simulink subsystem "Day4_5_Scenario_1"  (R2024a)
settings: Solver=VariableStepAuto  StartTime=0.0  StopTime=10.0  RelTol=1e-3
libraries: CarMaker4SL x29, robotalgslib x1, matrix_library x1, slpidlib x1
(part 1 of 2)
settings Model: Creator=junhyung.cha  LastModifiedBy=User

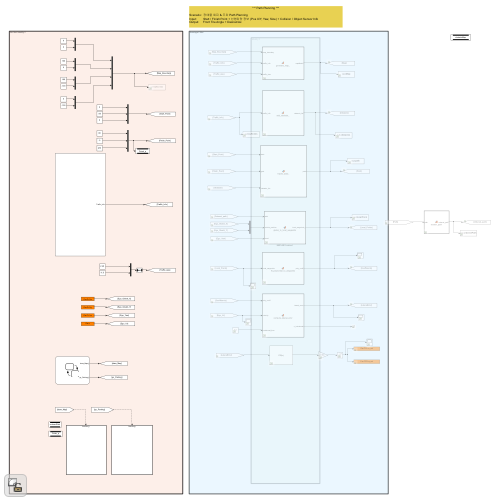
[thumbnail: Simulink's stored preview of the top-level diagram]
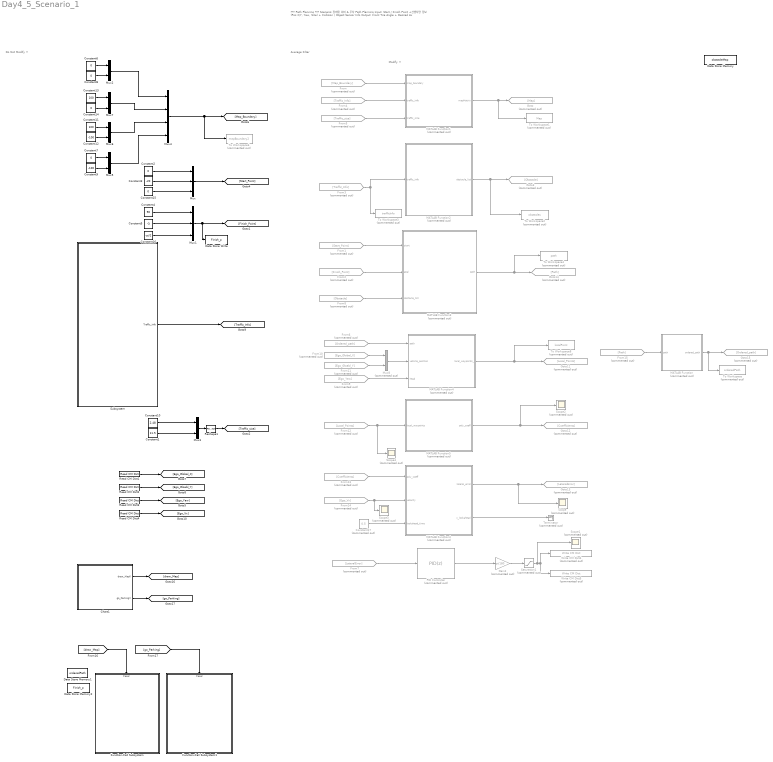
== system Day4_5_Scenario_1 ==
  note: Average Filter
  note: Do Not Modify !!
  note: Modify !!
  note: *** Path Planning ***
      |
      | Scenario: 장애물 회피 & 주차 Path Planning
      | Input: Start / Finish Point + 선행차량 정보 (Pos X/Y, Yaw, Size) + Collision / Object Sensor Info
      | Output: Front Tire Angle + Desired Ax
  Chart1 : Stateflow chart  TreatAsAtomicUnit=on
      settings: PortSchema="{\"entries\":[{\"content\":{\"sides\":[{\"content\":{},\"type\":\"ConnectorPlacement.EquallySpacedRectSide\",\"uuid\":\"919f2d59-559a-485a-ad64-4ca203985945\"},{\"content\":{\"connectorIds\":[\"Out2\",\"Out1\"],\"side\":\"RIGHT\"},\"type\":\"ConnectorPlacement.EquallySpacedRectSide\",\"uuid\":\"5a15d665-f3e4-404a-9c46-468f267f06f6\"},{\"content\":{\"side\":\"TOP\"},\"type\":\"ConnectorPlacement.EquallySpacedRectSide\",\"uuid\":\"06264e3b-ed7f-4ae7-832b-fa30ed2f7930\"}]},\"type\":\"ConnectorPlacement.EquallySpacedConnector\",\"uuid\":\"55c66715-cf4a-4d9b-b78f-cac3e631d511\"}],\"packageUris\":[\"http://schema.mathworks.com/mf0/Connector/R2020b\"],\"version\":\"1.0\"}"
  Constant1 : Constant  Value=11.5
  Constant10 : Constant  Value=2.48
  Constant11 : Constant  Value=100
  Constant12 : Constant  Value=-100
  Constant13 : Constant  Value=100
  Constant{2,6..8,14..15} (6 alike) : Constant  Value=0
  Constant16 : Constant  Value=-pi/2
  Constant17 : Constant  Commented=on  Value=0.5
  Constant3 : Constant  Value=-20
  Constant4 : Constant  Value=90
  Constant5 : Constant  Value=-3
  Constant9 : Constant  Value=-100
  Data Store Memory : DataStoreMemory  DataStoreName=obstacleMap  WriteAfterWriteMsg=warning  VectorParams1D=off  ShowAdditionalParam=off  Dimensions=[70 3]
  Data Store Memory1 : DataStoreMemory  DataStoreName=orderedPath  WriteAfterWriteMsg=warning  ShowAdditionalParam=off  Dimensions=[100 3]
  Data Store Memory2 : DataStoreMemory  DataStoreName=Finish_p  WriteAfterWriteMsg=warning  ShowAdditionalParam=off  Dimensions=[3 1]
  Data Store Write : DataStoreWrite  DataStoreName=Finish_p  IndexOptions=Index vector (dialog)  Indices=1  OutputSizes=1
  From : From  Commented=on  GotoTag=Map_Boundary
  From1 : From  Commented=on  GotoTag=Start_Point
  From10 : From  Commented=on  GotoTag=Ego_Global_X
  From11 : From  Commented=on  GotoTag=Ego_Gloabl_Y
  From12 : From  Commented=on  GotoTag=Local_Points
  From13 : From  Commented=on  GotoTag=Coefficients
  From14 : From  Commented=on  GotoTag=Ego_Vx
  From15 : From  Commented=on  GotoTag=Path
  From2 : From  Commented=on  GotoTag=Finish_Point
  From3 : From  Commented=on  GotoTag=Traffic_Info
  From4 : From  Commented=on  GotoTag=Traffic_Info
  From5 : From  Commented=on  GotoTag=Traffic_size
  From6 : From  Commented=on  GotoTag=Ordered_path
  From7 : From  Commented=on  GotoTag=LateralError
  From8 : From  Commented=on  GotoTag=Obstacle
  From9 : From  Commented=on  GotoTag=Ego_Yaw
  Function-Call Subsystem : Subsystem  TreatAsAtomicUnit=on
  Function-Call Subsystem1 : Subsystem  TreatAsAtomicUnit=on
  Gain2 : Gain  Commented=on  Gain=pi/180
  Goto : Goto  Commented=on  GotoTag=Map
  Goto11 : Goto  Commented=on  GotoTag=Local_Points
  Goto12 : Goto  Commented=on  GotoTag=Coefficients
  Goto13 : Goto  Commented=on  GotoTag=LateralError
  Goto14 : Goto  Commented=on  GotoTag=Path
  Goto15 : Goto  Commented=on  GotoTag=Ordered_path
  Goto3 : Goto  Commented=on  GotoTag=Obstacle
  MATLAB Function : MATLAB Function  Commented=on  TreatAsAtomicUnit=on
  MATLAB Function1 : MATLAB Function  Commented=on  TreatAsAtomicUnit=on
  MATLAB Function2 : MATLAB Function  Commented=on  TreatAsAtomicUnit=on
  MATLAB Function3 : MATLAB Function  Commented=on  TreatAsAtomicUnit=on
  MATLAB Function4 : MATLAB Function  Commented=on  TreatAsAtomicUnit=on
  "MATLAB Function4 " : MATLAB Function  Commented=on  TreatAsAtomicUnit=on
  MATLAB Function5 : MATLAB Function  Commented=on  TreatAsAtomicUnit=on
  Mux : Mux  Inputs=3
  Mux1 : Mux  Inputs=3
  Mux{2..3,5..7} (5 alike) : Mux  Inputs=2
  Mux4 : Mux
  Mux8 : Mux  Commented=on  Inputs=2
  PID Controller : slpidlib/PID Controller  Commented=on  Controller=PID  Form=Parallel  TimeDomain=Discrete-time  UseExternalTs=off  SampleTime=-1  IntegratorMethod=Forward Euler  FilterMethod=Forward Euler  ControllerParametersSource=internal  P=3  I=0  UseKiTs=off  D=0  UseExternalDerivativeSource=off  N=100  UseFilter=on  TunerSelectOption=Transfer Function Based (PID Tuner App)  InitialConditionSource=internal  InitialConditionForIntegrator=0  InitialConditionForFilter=0  DifferentiatorICPrevScaledInput=0  ExternalReset=none  TrackingMode=off  Kt=1  LimitOutput=off  SatLimitsSource=internal  UpperSaturationLimit=inf  LowerSaturationLimit=-inf  LinearizeAsGain=on  AntiWindupMode=none  Kb=1  LimitIntegrator=off  UpperIntegratorSaturationLimit=inf  LowerIntegratorSaturationLimit=-inf  POutMin=[]  POutMax=[]  IOutMin=[]  IOutMax=[]  DOutMin=[]  DOutMax=[]  NOutMin=[]  NOutMax=[]  SumOutMin=[]  SumOutMax=[]  SaturationOutMin=[]  SaturationOutMax=[]  PParamMin=[]  PParamMax=[]  IParamMin=[]  IParamMax=[]  DParamMin=[]  DParamMax=[]  NParamMin=[]  NParamMax=[]  KbParamMin=[]  KbParamMax=[]  KtParamMin=[]  KtParamMax=[]  KbOutMin=[]  KbOutMax=[]  KtOutMin=[]  KtOutMax=[]  IntegratorOutMin=[]  IntegratorOutMax=[]  FilterOutMin=[]  FilterOutMax=[]  SumI1OutMin=[]  SumI1OutMax=[]  SumI2OutMin=[]  SumI2OutMax=[]  SumI3OutMin=[]  SumI3OutMax=[]  SumI4OutMin=[]  SumI4OutMax=[]  SumDOutMin=[]  SumDOutMax=[]  DifferentiatorOutMin=[]  DifferentiatorOutMax=[]  FilterDiffOutCoefMin=[]  FilterDiffOutCoefMax=[]  ReciprocalOutMin=[]  ReciprocalOutMax=[]  SumDenOutMin=[]  SumDenOutMax=[]  SumNumOutMin=[]  SumNumOutMax=[]  DivideOutMin=[]  DivideOutMax=[]  UdiffTsProdOutMin=[]  UdiffTsProdOutMax=[]  NTsProdOutMin=[]  NTsProdOutMax=[]  UintegralTsProdOutMin=[]  UintegralTsProdOutMax=[]  UngainTsProdOutMin=[]  UngainTsProdOutMax=[]  ClampingZeroOutDataTypeStr=Inherit: Inherit via back propagation  ClampingZeroOutMin=[]  ClampingZeroOutMax=[]  FilterDenConstantOutDataTypeStr=Inherit: Inherit via back propagation  FilterDenConstantOutMin=[]  FilterDenConstantOutMax=[]  PCopyOutDataTypeStr=Inherit: Inherit via back propagation  PCopyOutMin=[]  PCopyOutMax=[]  NCopyOutDataTypeStr=Inherit: Inherit via back propagation  NCopyOutMin=[]  NCopyOutMax=[]  IntegratorContinuousStateAttributes=''  IntegratorStateMustResolveToSignalObject=off  IntegratorRTWStateStorageClass=Auto  FilterContinuousStateAttributes=''  FilterStateMustResolveToSignalObject=off  FilterRTWStateStorageClass=Auto  ParallelPVariant=InternalParameters  IdealPVariant=Disabled  IVariant=InternalParameters  DVariant=InternalParameters  IntegratorVariant=Discrete  SatVariant=Disabled  AWVariant=Passthrough  PCopyVariant=Disabled  TRVariant=Disabled  FdbkBlocksVariant=Forward  IdealPFdbkVariant=Disabled  SatFdbkVariant=Disabled  DerivativeFilterVariant=ForwardEulerFilter  NVariant=InternalParameters  NCopyVariant=Disabled  FilterICVariant=InternalICsFilter  IntegratorICVariant=InternalICs  ExternalResetVariant=Disabled  TRSumVariant=Passthrough  SumFdbkVariant=Disabled  SumVariant=Sum_PID  TsampFilterVariant=InternalTs  TsampNgainVariant=Passthrough  TsampIntegralVariant=Disabled_SignalSpec  ExternalSaturationOutDataTypeStr=Inherit: Same as second input  DerivativeSourceVariant=ErrorSignal
  Read CM Dict1 : CarMaker4SL/Read CM Dict  xname=Car.Fr1.tx  xsync=off  xstime=Inherited
  Read CM Dict2 : CarMaker4SL/Read CM Dict  xname=Car.Fr1.ty  xsync=off  xstime=Inherited
  Read CM Dict3 : CarMaker4SL/Read CM Dict  xname=Car.Fr1.rz  xsync=off  xstime=Inherited
  Read CM Dict4 : CarMaker4SL/Read CM Dict  xname=Car.v  xsync=off  xstime=Inherited
  Reshape1 : Reshape  OutputDimensionality=Row vector (2-D)  OutputDimensions=[2,2]
  Saturation1 : Saturate  Commented=on  UpperLimit=2  LowerLimit=-2
  Scope{,1..4} (5 alike) : Scope  Commented=on
  Subsystem : Subsystem
  Terminator : Terminator  Commented=on
  To Workspace : ToWorkspace  Commented=on  VariableName=orderedPath  SampleTime=-1
  To Workspace1 : ToWorkspace  Commented=on  VariableName=Map  SaveFormat=Timeseries  SampleTime=-1
  To Workspace2 : ToWorkspace  Commented=on  VariableName=obstacles  SampleTime=-1
  To Workspace3 : ToWorkspace  Commented=on  VariableName=trafficInfo  SaveFormat=Timeseries  SampleTime=-1
  To Workspace4 : ToWorkspace  Commented=on  VariableName=path  SampleTime=-1
  To Workspace6 : ToWorkspace  Commented=on  VariableName=mapBoundary2  SaveFormat=Timeseries  SampleTime=-1
  To Workspace8 : ToWorkspace  Commented=on  VariableName=localPoint  SampleTime=-1
  Write CM Dict4 : CarMaker4SL/Write CM Dict  Commented=on  xname=Car.CFL.rz_ext  xsync=off
  Write CM Dict5 : CarMaker4SL/Write CM Dict  Commented=on  xname=Car.CFR.rz_ext  xsync=off
  wires:
  Mux/1 -> [Start_Point]
  Constant2/1 -> Mux/1
  Constant3/1 -> Mux/2
  Constant5/1 -> Mux1/2
  Mux1/1 -> [Finish_Point], Data Store Write/1
  Constant4/1 -> Mux1/1
  Constant6/1 -> Mux2/1
  Constant8/1 -> Mux2/2
  Constant9/1 -> Mux5/2
  From/1 -> MATLAB Function1/1(map_boundary)
  Subsystem/1(Traffic_Info) -> [Traffic_Info]
  From3/1 -> MATLAB Function2/1(traffic_info), To Workspace3/1
  Mux3/1 -> Reshape1/1
  Constant10/1 -> Mux3/1
  Constant1/1 -> Mux3/2
  Mux2/1 -> Mux4/1
  Mux5/1 -> Mux4/4
  Mux4/1 -> [Map_Boundary], To Workspace6/1
  Constant7/1 -> Mux5/1
  From4/1 -> MATLAB Function1/2(traffic_info)
  From5/1 -> MATLAB Function1/3(traffic_size)
  Reshape1/1 -> [Traffic_size]
  MATLAB Function1/1(mapMatrix) -> Goto/1, To Workspace1/1
  Read CM Dict4/1 -> [Ego_Vx]
  Read CM Dict1/1 -> [Ego_Global_X]
  Read CM Dict2/1 -> [Ego_Gloabl_Y]
  Read CM Dict3/1 -> [Ego_Yaw]
  Constant11/1 -> Mux6/1
  Constant12/1 -> Mux6/2
  Constant13/1 -> Mux7/1
  Constant14/1 -> Mux7/2
  Mux7/1 -> Mux4/2
  Mux6/1 -> Mux4/3
  Constant15/1 -> Mux/3
  Constant16/1 -> Mux1/3
  MATLAB Function2/1(obstacle_list) -> Goto3/1, To Workspace2/1
  From1/1 -> MATLAB Function3/1(start)
  From2/1 -> MATLAB Function3/2(goal)
  From8/1 -> MATLAB Function3/3(obstacle_list)
  Constant17/1 -> MATLAB Function4/3(lookahead_time)
  From7/1 -> PID Controller/1
  Gain2/1 -> Saturation1/1
  From11/1 -> Mux8/2
  Saturation1/1 -> Write CM Dict4/1, Write CM Dict5/1, Scope1/1
  Mux8/1 -> "MATLAB Function4 "/2(vehicle_position)
  From13/1 -> MATLAB Function4/1(poly_coeff)
  MATLAB Function5/1(poly_coeff) -> Goto12/1, Scope2/1
  MATLAB Function4/1(lateral_error) -> Goto13/1, Scope/1
  MATLAB Function4/2(x_lookahead) -> Terminator/1
  From9/1 -> "MATLAB Function4 "/3(head)
  From12/1 -> MATLAB Function5/1(local_waypoints), Scope4/1
  From10/1 -> Mux8/1
  "MATLAB Function4 "/1(local_waypoints_) -> Goto11/1, To Workspace8/1
  From6/1 -> "MATLAB Function4 "/1(path)
  From14/1 -> MATLAB Function4/2(velocity), Scope3/1
  PID Controller/1 -> Gain2/1
  MATLAB Function3/1(path) -> Goto14/1, To Workspace4/1
  From15/1 -> MATLAB Function/1(path)
  MATLAB Function/1(ordered_path) -> Goto15/1, To Workspace/1
  Chart1/2(draw_Map()) -> [draw_Map]
  [draw_Map] -> Function-Call Subsystem/Trigger
  Chart1/1(go_Parking()) -> [go_Parking]
  [go_Parking] -> Function-Call Subsystem1/Trigger

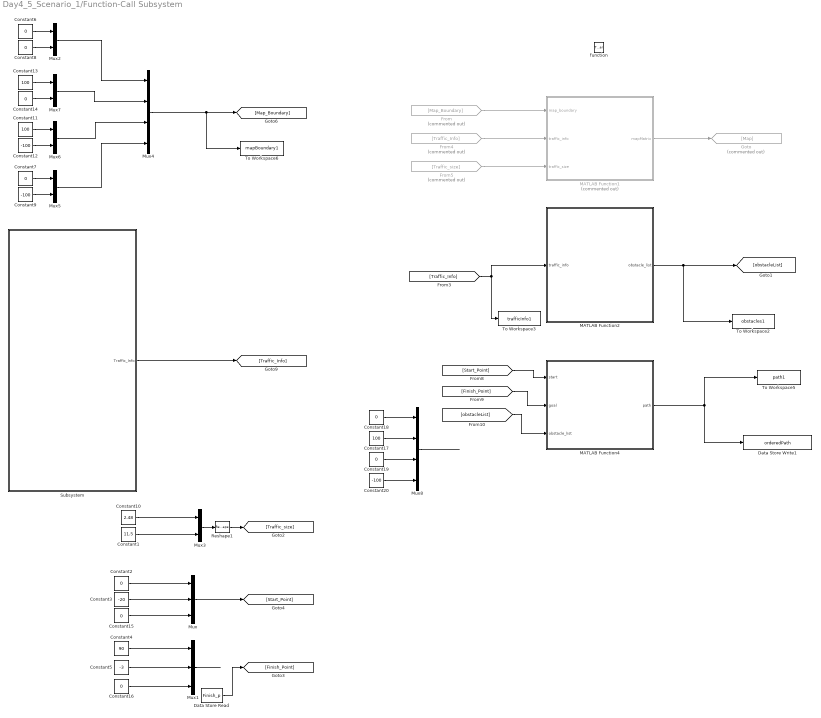
== system Day4_5_Scenario_1/Function-Call Subsystem ==
  function : TriggerPort  TriggerType=function-call  VariantControl=(inherit)
  Constant1 : Constant  Value=11.5
  Constant10 : Constant  Value=2.48
  Constant11 : Constant  Value=100
  Constant12 : Constant  Value=-100
  Constant13 : Constant  Value=100
  Constant{2,6..8,14..16,18..19} (9 alike) : Constant  Value=0
  Constant17 : Constant  Value=100
  Constant20 : Constant  Value=-100
  Constant3 : Constant  Value=-20
  Constant4 : Constant  Value=90
  Constant5 : Constant  Value=-3
  Constant9 : Constant  Value=-100
  Data Store Read : DataStoreRead  DataStoreName=Finish_p  IndexOptions=Index vector (dialog)  Indices=1  OutputSizes=1
  Data Store Write1 : DataStoreWrite  DataStoreName=orderedPath  IndexOptions=Index vector (dialog)  Indices=1  OutputSizes=1
  From : From  Commented=on  GotoTag=Map_Boundary
  From4 : From  Commented=on  GotoTag=Traffic_Info
  From5 : From  Commented=on  GotoTag=Traffic_size
  Goto : Goto  Commented=on  GotoTag=Map
  MATLAB Function1 : MATLAB Function  Commented=on  TreatAsAtomicUnit=on
  MATLAB Function2 : MATLAB Function  TreatAsAtomicUnit=on
  MATLAB Function4 : MATLAB Function  TreatAsAtomicUnit=on
  Mux : Mux  Inputs=3
  Mux1 : Mux  Inputs=3
  Mux{2..3,5..7} (5 alike) : Mux  Inputs=2
  Mux4 : Mux
  Mux8 : Mux
  Reshape1 : Reshape  OutputDimensionality=Row vector (2-D)  OutputDimensions=[2,2]
  Subsystem : Subsystem
  To Workspace2 : ToWorkspace  VariableName=obstacles1  SampleTime=-1
  To Workspace3 : ToWorkspace  VariableName=trafficInfo1  SaveFormat=Timeseries  SampleTime=-1
  To Workspace5 : ToWorkspace  VariableName=path1  SampleTime=-1
      settings: Save2DSignal=2-D array (concatenate along first dimension)
  To Workspace6 : ToWorkspace  VariableName=mapBoundary1  SampleTime=-1
  wires:
  MATLAB Function4/1(path) -> To Workspace5/1, Data Store Write1/1
  Mux8/1 -> ?
  Constant17/1 -> Mux8/2
  Constant18/1 -> Mux8/1
  Constant20/1 -> Mux8/4
  Constant19/1 -> Mux8/3
  [obstacleList] -> MATLAB Function4/3(obstacle_list)
  [Finish_Point] -> MATLAB Function4/2(goal)
  [Start_Point] -> MATLAB Function4/1(start)
  Data Store Read/1 -> [Finish_Point]
  Mux1/1 -> ?
  Constant3/1 -> Mux/2
  Mux/1 -> [Start_Point]
  Constant15/1 -> Mux/3
  Constant5/1 -> Mux1/2
  Constant4/1 -> Mux1/1
  Constant2/1 -> Mux/1
  Constant16/1 -> Mux1/3
  Constant12/1 -> Mux6/2
  MATLAB Function2/1(obstacle_list) -> [obstacleList], To Workspace2/1
  Subsystem/1(Traffic_Info) -> [Traffic_Info]
  Mux5/1 -> Mux4/4
  Mux4/1 -> [Map_Boundary], To Workspace6/1
  [Traffic_Info] -> MATLAB Function2/1(traffic_info), To Workspace3/1
  Constant13/1 -> Mux7/1
  Reshape1/1 -> [Traffic_size]
  Constant1/1 -> Mux3/2
  Constant6/1 -> Mux2/1
  Constant8/1 -> Mux2/2
  From5/1 -> MATLAB Function1/3(traffic_size)
  Constant10/1 -> Mux3/1
  From4/1 -> MATLAB Function1/2(traffic_info)
  Mux6/1 -> Mux4/3
  From/1 -> MATLAB Function1/1(map_boundary)
  Mux3/1 -> Reshape1/1
  Constant7/1 -> Mux5/1
  Constant14/1 -> Mux7/2
  Constant11/1 -> Mux6/1
  Mux2/1 -> Mux4/1
  Mux7/1 -> Mux4/2
  MATLAB Function1/1(mapMatrix) -> Goto/1
  Constant9/1 -> Mux5/2

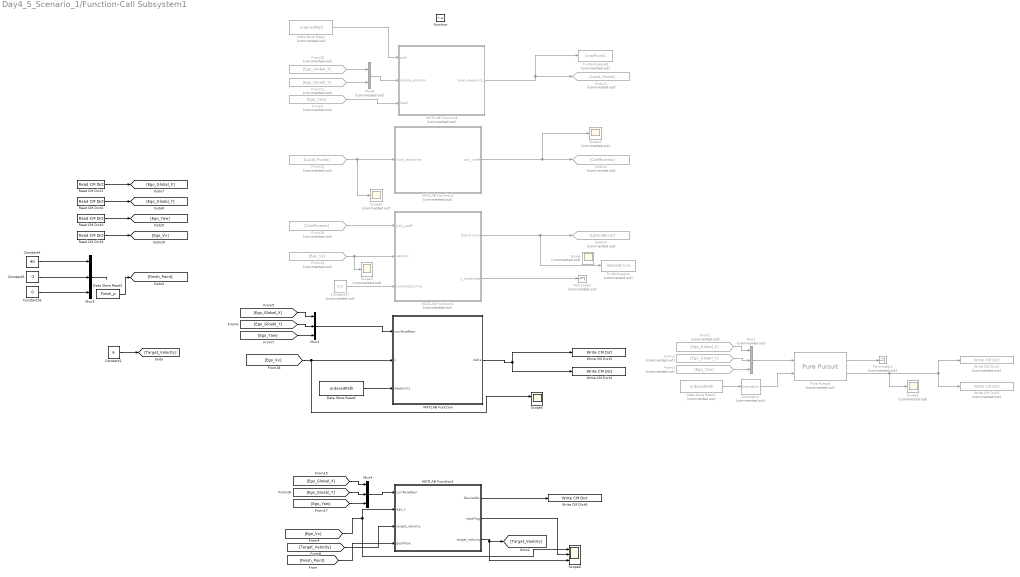
== system Day4_5_Scenario_1/Function-Call Subsystem1 ==
  function : TriggerPort  TriggerType=function-call  VariantControl=(inherit)
  Constant1 : Constant  Value=6
  Constant16 : Constant  Value=0
  Constant17 : Constant  Commented=on  Value=0.5
  Constant4 : Constant  Value=90
  Constant5 : Constant  Value=-3
  Data Store Read : DataStoreRead  Commented=on  DataStoreName=orderedPath  IndexOptions=Index vector (dialog)  Indices=1  OutputSizes=1
  Data Store Read1 : DataStoreRead  Commented=on  DataStoreName=orderedPath  IndexOptions=Index vector (dialog)  Indices=1  OutputSizes=1
  Data Store Read2 : DataStoreRead  DataStoreName=orderedPath  IndexOptions=Index vector (dialog)  Indices=1  OutputSizes=1
  Data Store Read3 : DataStoreRead  DataStoreName=Finish_p  IndexOptions=Index vector (dialog)  Indices=1  OutputSizes=1
  From1 : From  Commented=on  GotoTag=Ego_Global_X
  From10 : From  Commented=on  GotoTag=Ego_Global_X
  From11 : From  Commented=on  GotoTag=Ego_Gloabl_Y
  From12 : From  Commented=on  GotoTag=Local_Points
  From13 : From  Commented=on  GotoTag=Coefficients
  From14 : From  Commented=on  GotoTag=Ego_Vx
  From2 : From  Commented=on  GotoTag=Ego_Gloabl_Y
  From3 : From  Commented=on  GotoTag=Ego_Yaw
  From9 : From  Commented=on  GotoTag=Ego_Yaw
  Goto11 : Goto  Commented=on  GotoTag=Local_Points
  Goto12 : Goto  Commented=on  GotoTag=Coefficients
  Goto13 : Goto  Commented=on  GotoTag=LateralError
  MATLAB Function : MATLAB Function  TreatAsAtomicUnit=on
  MATLAB Function2 : MATLAB Function  TreatAsAtomicUnit=on
  MATLAB Function4 : MATLAB Function  Commented=on  TreatAsAtomicUnit=on
  "MATLAB Function4 " : MATLAB Function  Commented=on  TreatAsAtomicUnit=on
  MATLAB Function5 : MATLAB Function  Commented=on  TreatAsAtomicUnit=on
  Mux1 : Mux  Commented=on  Inputs=3
  Mux2 : Mux  Inputs=3
  Mux3 : Mux  Inputs=3
  Mux4 : Mux  Inputs=3
  Mux8 : Mux  Commented=on  Inputs=2
  Pure Pursuit : robotalgslib/Pure Pursuit  Commented=on  DesiredLinearVelocityPort=off  DesiredLinearVelocity=5  MaxAngularVelocity=2.0  LookaheadDistancePort=off  LookaheadDistance=3  TargetDirPort=off  SimulateUsing=Code generation
  Read CM Dict1 : CarMaker4SL/Read CM Dict  xname=Car.Fr1.tx  xsync=off  xstime=Inherited
  Read CM Dict2 : CarMaker4SL/Read CM Dict  xname=Car.Fr1.ty  xsync=off  xstime=Inherited
  Read CM Dict3 : CarMaker4SL/Read CM Dict  xname=Car.Fr1.rz  xsync=off  xstime=Inherited
  Read CM Dict4 : CarMaker4SL/Read CM Dict  xname=Car.v  xsync=off  xstime=Inherited
  Scope{,1..4} (5 alike) : Scope  Commented=on
  Scope5 : Scope  NumInputPorts=2
  Scope6 : Scope  NumInputPorts=3
  Submatrix : matrix_library/Submatrix  Commented=on  RowSpan=Range of rows  RowStartMode=First  RowStartIndex=1  RowEndMode=Last  RowEndIndex=1  ColSpan=Range of columns  ColStartMode=First  ColStartIndex=1  ColEndMode=Index  ColEndIndex=2
  Terminator : Terminator  Commented=on
  Terminator1 : Terminator  Commented=on
  To Workspace : ToWorkspace  Commented=on  VariableName=lateralErrors  SampleTime=-1
      settings: Save2DSignal=2-D array (concatenate along first dimension)
  To Workspace8 : ToWorkspace  Commented=on  VariableName=localPoint1  SampleTime=-1
  Write CM Dict1 : CarMaker4SL/Write CM Dict  Commented=on  xname=Car.CFL.rz_ext  xsync=off
  Write CM Dict2 : CarMaker4SL/Write CM Dict  Commented=on  xname=Car.CFR.rz_ext  xsync=off
  Write CM Dict3 : CarMaker4SL/Write CM Dict  xname=Car.CFL.rz_ext  xsync=off
  Write CM Dict4 : CarMaker4SL/Write CM Dict  xname=Car.CFR.rz_ext  xsync=off
  Write CM Dict6 : CarMaker4SL/Write CM Dict  xname=AccelCtrl.DesiredAx  xsync=off
  wires:
  Data Store Read3/1 -> [Finish_Point]
  [Ego_Vx] -> MATLAB Function/2(v), Scope5/1
  MATLAB Function2/3(target_velocity) -> [Target_Veolcity], Scope6/3
  [Ego_Yaw] -> Mux4/3
  [Ego_Global_X] -> Mux4/1
  [Ego_Gloabl_Y] -> Mux4/2
  Mux4/1 -> MATLAB Function2/1(currPoseRear)
  MATLAB Function2/2(stopFlag) -> Scope6/2
  Constant1/1 -> [Target_Velocity]
  MATLAB Function2/1(DesiredAx) -> Write CM Dict6/1
  [Ego_Vx] -> MATLAB Function2/2(ego_v), Scope6/1
  [Target_Velocity] -> MATLAB Function2/3("target_velocity ")
  [Finish_Point] -> MATLAB Function2/4(goalPose)
  Constant16/1 -> Mux3/3
  Constant4/1 -> Mux3/1
  Constant5/1 -> Mux3/2
  Mux3/1 -> ?
  Data Store Read2/1 -> MATLAB Function/3(waypoints)
  [Ego_Global_X] -> Mux2/1
  Mux2/1 -> MATLAB Function/1(currPoseRear)
  [Ego_Yaw] -> Mux2/3
  [Ego_Gloabl_Y] -> Mux2/2
  MATLAB Function/1(delta) -> Write CM Dict4/1, Write CM Dict3/1
  Submatrix/1 -> Pure Pursuit/2
  Data Store Read1/1 -> Submatrix/1
  Pure Pursuit/2 -> Write CM Dict2/1, Write CM Dict1/1, Scope1/1
  Pure Pursuit/1 -> Terminator1/1
  From1/1 -> Mux1/1
  From2/1 -> Mux1/2
  From3/1 -> Mux1/3
  Mux1/1 -> Pure Pursuit/1
  Data Store Read/1 -> "MATLAB Function4 "/1(path)
  Read CM Dict2/1 -> [Ego_Gloabl_Y]
  MATLAB Function5/1(poly_coeff) -> Goto12/1, Scope2/1
  Read CM Dict1/1 -> [Ego_Global_X]
  Read CM Dict3/1 -> [Ego_Yaw]
  Read CM Dict4/1 -> [Ego_Vx]
  Mux8/1 -> "MATLAB Function4 "/2(vehicle_position)
  From14/1 -> MATLAB Function4/2(velocity), Scope3/1
  From11/1 -> Mux8/2
  From13/1 -> MATLAB Function4/1(poly_coeff)
  MATLAB Function4/2(x_lookahead) -> Terminator/1
  Constant17/1 -> MATLAB Function4/3(lookahead_time)
  "MATLAB Function4 "/1(local_waypoints_) -> Goto11/1, To Workspace8/1
  From10/1 -> Mux8/1
  From9/1 -> "MATLAB Function4 "/3(head)
  MATLAB Function4/1(lateral_error) -> Goto13/1, To Workspace/1
  From12/1 -> MATLAB Function5/1(local_waypoints), Scope4/1

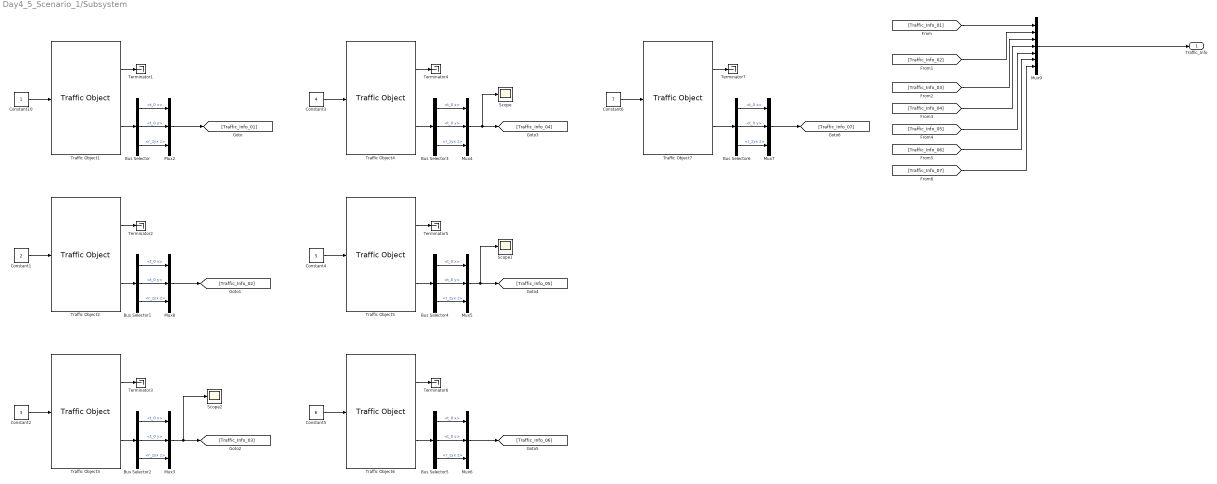
== system Day4_5_Scenario_1/Subsystem ==
  Bus Selector{,1..6} (7 alike) : BusSelector  OutputSignals=t_0 x,t_0 y,r_zyx z
  Constant1 : Constant  Value=2
  Constant10 : Constant
  Constant2 : Constant  Value=3
  Constant3 : Constant  Value=4
  Constant4 : Constant  Value=5
  Constant5 : Constant  Value=6
  Constant6 : Constant  Value=7
  Mux{2..8} (7 alike) : Mux  Inputs=3
  Mux9 : Mux  Inputs=7
  Scope : Scope
  Scope1 : Scope
  Scope2 : Scope
  Terminator{1..7} (7 alike) : Terminator
  Traffic Object1 : CarMaker4SL/Traffic Object  xname=T01  ximode=Traffic Id  xstime=Inherited
      settings: SourceProductName=CarMaker4SL
  Traffic Object2 : CarMaker4SL/Traffic Object  xname=T02  ximode=Traffic Id  xstime=Inherited
      settings: SourceProductName=CarMaker4SL
  Traffic Object3 : CarMaker4SL/Traffic Object  xname=T03  ximode=Traffic Id  xstime=Inherited
      settings: SourceProductName=CarMaker4SL
  Traffic Object4 : CarMaker4SL/Traffic Object  xname=T04  ximode=Traffic Id  xstime=Inherited
      settings: SourceProductName=CarMaker4SL
  Traffic Object5 : CarMaker4SL/Traffic Object  xname=T05  ximode=Traffic Id  xstime=Inherited
      settings: SourceProductName=CarMaker4SL
  Traffic Object6 : CarMaker4SL/Traffic Object  xname=T06  ximode=Traffic Id  xstime=Inherited
      settings: SourceProductName=CarMaker4SL
  Traffic Object7 : CarMaker4SL/Traffic Object  xname=T07  ximode=Traffic Id  xstime=Inherited
      settings: SourceProductName=CarMaker4SL
  Traffic_Info : Outport
  wires:
  [Traffic_Info_07] -> Mux9/7
  [Traffic_Info_06] -> Mux9/6
  [Traffic_Info_05] -> Mux9/5
  [Traffic_Info_04] -> Mux9/4
  [Traffic_Info_03] -> Mux9/3
  Mux9/1 -> Traffic_Info/1
  [Traffic_Info_02] -> Mux9/2
  [Traffic_Info_01] -> Mux9/1
  Mux2/1 -> [Traffic_Info_01]
  Traffic Object7/2 -> Bus Selector6/1
  Bus Selector6/3 -> Mux7/3  "<r_zyx z>"
  Bus Selector6/1 -> Mux7/1  "<t_0 x>"
  Mux7/1 -> [Traffic_Info_07]
  Bus Selector6/2 -> Mux7/2  "<t_0 y>"
  Traffic Object6/2 -> Bus Selector5/1
  Bus Selector5/3 -> Mux6/3  "<r_zyx z>"
  Bus Selector5/1 -> Mux6/1  "<t_0 x>"
  Mux6/1 -> [Traffic_Info_06]
  Bus Selector5/2 -> Mux6/2  "<t_0 y>"
  Traffic Object5/2 -> Bus Selector4/1
  Bus Selector4/3 -> Mux5/3  "<r_zyx z>"
  Bus Selector4/1 -> Mux5/1  "<t_0 x>"
  Mux5/1 -> [Traffic_Info_05], Scope1/1
  Bus Selector4/2 -> Mux5/2  "<t_0 y>"
  Traffic Object4/2 -> Bus Selector3/1
  Bus Selector3/3 -> Mux4/3  "<r_zyx z>"
  Bus Selector3/1 -> Mux4/1  "<t_0 x>"
  Mux4/1 -> [Traffic_Info_04], Scope/1
  Bus Selector3/2 -> Mux4/2  "<t_0 y>"
  Traffic Object3/2 -> Bus Selector2/1
  Bus Selector2/3 -> Mux3/3  "<r_zyx z>"
  Bus Selector2/1 -> Mux3/1  "<t_0 x>"
  Mux3/1 -> [Traffic_Info_03], Scope2/1
  Bus Selector2/2 -> Mux3/2  "<t_0 y>"
  Traffic Object2/2 -> Bus Selector1/1
  Bus Selector1/3 -> Mux8/3  "<r_zyx z>"
  Bus Selector1/1 -> Mux8/1  "<t_0 x>"
  Mux8/1 -> [Traffic_Info_02]
  Bus Selector1/2 -> Mux8/2  "<t_0 y>"
  Bus Selector/3 -> Mux2/3  "<r_zyx z>"
  Bus Selector/2 -> Mux2/2  "<t_0 y>"
  Bus Selector/1 -> Mux2/1  "<t_0 x>"
  Traffic Object1/2 -> Bus Selector/1
  Traffic Object7/1 -> Terminator7/1
  Constant6/1 -> Traffic Object7/1
  Constant5/1 -> Traffic Object6/1
  Traffic Object6/1 -> Terminator6/1
  Traffic Object5/1 -> Terminator5/1
  Constant4/1 -> Traffic Object5/1
  Constant3/1 -> Traffic Object4/1
  Traffic Object4/1 -> Terminator4/1
  Traffic Object3/1 -> Terminator3/1
  Constant2/1 -> Traffic Object3/1
  Constant1/1 -> Traffic Object2/1
  Traffic Object2/1 -> Terminator2/1
  Traffic Object1/1 -> Terminator1/1
  Constant10/1 -> Traffic Object1/1

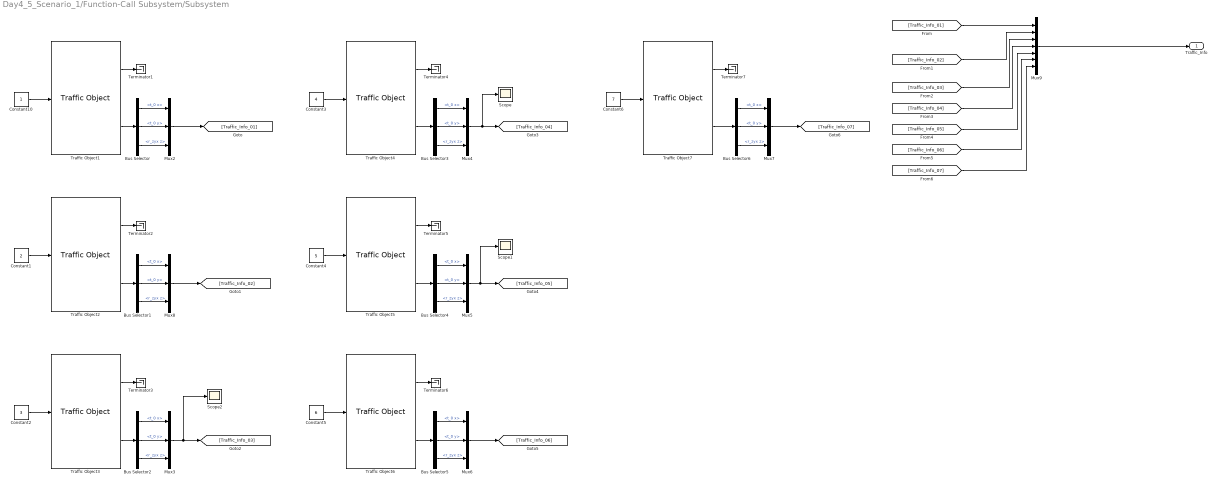
== system Day4_5_Scenario_1/Function-Call Subsystem/Subsystem ==
  Bus Selector{,1..6} (7 alike) : BusSelector  OutputSignals=t_0 x,t_0 y,r_zyx z
  Constant1 : Constant  Value=2
  Constant10 : Constant
  Constant2 : Constant  Value=3
  Constant3 : Constant  Value=4
  Constant4 : Constant  Value=5
  Constant5 : Constant  Value=6
  Constant6 : Constant  Value=7
  Mux{2..8} (7 alike) : Mux  Inputs=3
  Mux9 : Mux  Inputs=7
  Scope : Scope
  Scope1 : Scope
  Scope2 : Scope
  Terminator{1..7} (7 alike) : Terminator
  Traffic Object1 : CarMaker4SL/Traffic Object  xname=T01  ximode=Traffic Id  xstime=Inherited
      settings: SourceProductName=CarMaker4SL
  Traffic Object2 : CarMaker4SL/Traffic Object  xname=T02  ximode=Traffic Id  xstime=Inherited
      settings: SourceProductName=CarMaker4SL
  Traffic Object3 : CarMaker4SL/Traffic Object  xname=T03  ximode=Traffic Id  xstime=Inherited
      settings: SourceProductName=CarMaker4SL
  Traffic Object4 : CarMaker4SL/Traffic Object  xname=T04  ximode=Traffic Id  xstime=Inherited
      settings: SourceProductName=CarMaker4SL
  Traffic Object5 : CarMaker4SL/Traffic Object  xname=T05  ximode=Traffic Id  xstime=Inherited
      settings: SourceProductName=CarMaker4SL
  Traffic Object6 : CarMaker4SL/Traffic Object  xname=T06  ximode=Traffic Id  xstime=Inherited
      settings: SourceProductName=CarMaker4SL
  Traffic Object7 : CarMaker4SL/Traffic Object  xname=T07  ximode=Traffic Id  xstime=Inherited
      settings: SourceProductName=CarMaker4SL
  Traffic_Info : Outport
  wires:
  [Traffic_Info_07] -> Mux9/7
  [Traffic_Info_06] -> Mux9/6
  [Traffic_Info_05] -> Mux9/5
  [Traffic_Info_04] -> Mux9/4
  [Traffic_Info_03] -> Mux9/3
  Mux9/1 -> Traffic_Info/1
  [Traffic_Info_02] -> Mux9/2
  [Traffic_Info_01] -> Mux9/1
  Mux2/1 -> [Traffic_Info_01]
  Traffic Object7/2 -> Bus Selector6/1
  Bus Selector6/3 -> Mux7/3  "<r_zyx z>"
  Bus Selector6/1 -> Mux7/1  "<t_0 x>"
  Mux7/1 -> [Traffic_Info_07]
  Bus Selector6/2 -> Mux7/2  "<t_0 y>"
  Traffic Object6/2 -> Bus Selector5/1
  Bus Selector5/3 -> Mux6/3  "<r_zyx z>"
  Bus Selector5/1 -> Mux6/1  "<t_0 x>"
  Mux6/1 -> [Traffic_Info_06]
  Bus Selector5/2 -> Mux6/2  "<t_0 y>"
  Traffic Object5/2 -> Bus Selector4/1
  Bus Selector4/3 -> Mux5/3  "<r_zyx z>"
  Bus Selector4/1 -> Mux5/1  "<t_0 x>"
  Mux5/1 -> [Traffic_Info_05], Scope1/1
  Bus Selector4/2 -> Mux5/2  "<t_0 y>"
  Traffic Object4/2 -> Bus Selector3/1
  Bus Selector3/3 -> Mux4/3  "<r_zyx z>"
  Bus Selector3/1 -> Mux4/1  "<t_0 x>"
  Mux4/1 -> [Traffic_Info_04], Scope/1
  Bus Selector3/2 -> Mux4/2  "<t_0 y>"
  Traffic Object3/2 -> Bus Selector2/1
  Bus Selector2/3 -> Mux3/3  "<r_zyx z>"
  Bus Selector2/1 -> Mux3/1  "<t_0 x>"
  Mux3/1 -> [Traffic_Info_03], Scope2/1
  Bus Selector2/2 -> Mux3/2  "<t_0 y>"
  Traffic Object2/2 -> Bus Selector1/1
  Bus Selector1/3 -> Mux8/3  "<r_zyx z>"
  Bus Selector1/1 -> Mux8/1  "<t_0 x>"
  Mux8/1 -> [Traffic_Info_02]
  Bus Selector1/2 -> Mux8/2  "<t_0 y>"
  Bus Selector/3 -> Mux2/3  "<r_zyx z>"
  Bus Selector/2 -> Mux2/2  "<t_0 y>"
  Bus Selector/1 -> Mux2/1  "<t_0 x>"
  Traffic Object1/2 -> Bus Selector/1
  Traffic Object7/1 -> Terminator7/1
  Constant6/1 -> Traffic Object7/1
  Constant5/1 -> Traffic Object6/1
  Traffic Object6/1 -> Terminator6/1
  Traffic Object5/1 -> Terminator5/1
  Constant4/1 -> Traffic Object5/1
  Constant3/1 -> Traffic Object4/1
  Traffic Object4/1 -> Terminator4/1
  Traffic Object3/1 -> Terminator3/1
  Constant2/1 -> Traffic Object3/1
  Constant1/1 -> Traffic Object2/1
  Traffic Object2/1 -> Terminator2/1
  Traffic Object1/1 -> Terminator1/1
  Constant10/1 -> Traffic Object1/1

== matlab function Day4_5_Scenario_1/Function-Call Subsystem/MATLAB Function2 ==
  settings: sampleTime=0.1
  data: traffic_info input; obstacle_list output
function obstacle_list = add_obstacle_(traffic_info)
    % 차량 사이즈
    car_w = 2.48;            % 전폭
    car_l = 11.5;            % 전장

    % 장애물 파라미터
    r = car_w / 2 + 2;       % 각 원의 반지름 (1.24 + 2)
    n_circles = 5;          % 각 차량당 원 개수
    interval = car_l / n_circles;  % 원 간격

    % 최대 장애물 개수
    max_obs = 100;
    obstacle_list = zeros(max_obs, 3);  % [x, y, r]

    % === 데이터 복원 ===
    % 데이터가 직렬화된 벡터 형태로 들어오는 경우 처리
    if size(traffic_info, 2) == 1
        % 데이터를 3열 형태로 변환
        n = length(traffic_info) / 3;
        if mod(length(traffic_info), 3) == 0
            % 직렬 데이터를 [N x 3] 행렬로 변환
            latest_data = reshape(traffic_info, 3, n)';  % [N x 3]
            %disp('Reconstructed Data:');
            %disp(latest_data);  % 디버그 출력
        else
            warning('Invalid data length for traffic_info');
            return;
        end
    else
        latest_data = traffic_info;
    end

    % === 데이터 유효성 검사 ===
    if isempty(latest_data) || size(latest_data, 2) < 3
        warning('Latest data is empty or has incorrect dimensions');
        return;
    end

    % 중복 제거: unique 함수 사용 가능 여부 확인
    if size(latest_data, 1) > 1
        % unique 함수로 중복 좌표 제거
        [~, unique_indices] = unique(latest_data(:, 1:2), 'rows', 'stable');
        unique_data = latest_data(unique_indices, :);
    else
        % 데이터가 하나만 있는 경우 그대로 사용
        unique_data = latest_data;
    end

    % 입력 데이터 유효성 검사 및 reshape 처리
    unique_data = reshape(unique_data, [], 3);  % [N x 3]
    [n_rows, ~] = size(unique_data);

    % 장애물 좌표 생성
    count = 0;
    for i = 1:n_rows
        x_head = unique_data(i, 1);
        y_head = unique_data(i, 2);
        yaw = unique_data(i, 3);  % 각도(rad)

        % Yaw 값 검증
        if isnan(yaw) || ~isfinite(yaw)
            yaw = 0;
        end

        % 장애물 생성 (차량의 길이 방향으로)
        for j = 0:n_circles-1
            dx = cos(yaw) * (j * interval);
            dy = sin(yaw) * (j * interval);
            xc = x_head + dx;
            yc = y_head + dy;

            count = count + 1;
            if count <= max_obs
                obstacle_list(count, :) = [xc, yc, r];
            else
                break;
            end
        end
    end

    % 디버그: 결과 확인
    %disp('Generated Obstacle List:');
    %disp(obstacle_list);
    disp("generate_Map_Finish");
end

== matlab function Day4_5_Scenario_1/MATLAB Function ==
  data: path input; ordered_path output
function ordered_path = reorder_path(path)
    %#codegen
    % 입력: path (100x3) - 역순 경로
    % 출력: ordered_path (100x3) - 정순 경로

    % 고정 크기 배열 선언 (100x3)
    ordered_path = NaN(100, 3);  
    
    % 유효 경로 필터링 (NaN 값 제거)
    valid_idx = ~isnan(path(:, 1)) & ~isnan(path(:, 2)) & ~isnan(path(:, 3));
    valid_path = path(valid_idx, :);

    % 유효 경로 개수
    num_points = size(valid_path, 1);

    % 역순으로 배열 채우기 (고정 크기 유지)
    for i = 1:num_points
        ordered_path(i, :) = valid_path(num_points - i + 1, :);
    end

    % 나머지 부분 NaN으로 채우기
    if num_points < 100
        ordered_path((num_points+1):100, :) = NaN;
    end
end

== matlab function Day4_5_Scenario_1/MATLAB Function1 ==
  settings: sampleTime=0.05
  data: map_boundary input; mapMatrix output size=[1000, 1000]; traffic_info input; traffic_size input
% map_boundary = [0, 0, 100, 0, 100, -100, 0, -100];  % 시계방향 사각형
% traffic_info = [
%     40   -12   pi/2;
%     40   -24   pi/2;
%     40   -36   pi/2;
%     40   -48   pi/2;
%     39   -50   0;
%     51   -50   0;
%     63   -50   0];  % [x_head, y_head, yaw]
% traffic_size = [2.48, 11.5];    % [width, length] (m)
% start_point  = [0, -20];
% finish_point = [80, -3];
% 
% a = generate_map_(map_boundary, traffic_info, traffic_size);

function mapMatrix = generate_map_(map_boundary, traffic_info, traffic_size)
%#codegen
% 맵 바운더리 + 장애물 테두리를 마스킹하는 함수
% Y축 반전 처리만 적용 (Y는 -100~0 → mapMatrix는 1~100)

    % === 초기화 ===
    mapMatrix = zeros(100, 100);

    % === reshape 및 파라미터 ===
    traffic_info = reshape(traffic_info, [], 3);  % [N x 3]
    num_traffic = size(traffic_info, 1);
    width  = traffic_size(1);
    length = traffic_size(2);

    % === 장애물 테두리 처리 ===
    for i = 1:num_traffic
        x_head = traffic_info(i,1);
        y_head = traffic_info(i,2);
        yaw    = traffic_info(i,3);
       
        % 머리 좌표를 중심 기준으로 사용
        xc = x_head;
        yc = y_head;

        dx = width / 2;
        dy = length;
        local = [
            0, -dx;
            0,  dx;
            dy, dx;
            dy, -dx
        ];

        R = [cos(yaw), -sin(yaw); sin(yaw), cos(yaw)];
        global_pts = zeros(5, 2);  % 4개 꼭짓점 + 첫 점
        
        global_pts(1:4, :) = (R * local')' + [xc, yc];
        global_pts(5, :)   = global_pts(1, :);  % 꼭짓점 닫기

        for k = 1:4
            x1 = global_pts(k,1);   y1 = global_pts(k,2);
            x2 = global_pts(k+1,1); y2 = global_pts(k+1,2);
            N = 100;
            xs = linspace(x1, x2, N);
            ys = linspace(y1, y2, N);
            for j = 1:N
                x_idx = round(xs(j));
                y_idx = round(-ys(j));  % ✅ Y 좌표 반전

                % 인덱스 클리핑
                x_idx = min(max(x_idx, 1), 100);
                y_idx = min(max(y_idx, 1), 100);

                mapMatrix(y_idx, x_idx) = 1;
            end
        end
    end

    % === 바운더리 테두리 처리 ===
    xb = map_boundary(1:2:end);
    yb = map_boundary(2:2:end);
    xb(end+1) = xb(1);
    yb(end+1) = yb(1);
    for k = 1:4
        x1 = xb(k);   y1 = yb(k);
        x2 = xb(k+1); y2 = yb(k+1);
        N = 100;
        xs = linspace(x1, x2, N);
        ys = linspace(y1, y2, N);
        for j = 1:N
            x_idx = round(xs(j));
            y_idx = round(-ys(j));  % ✅ Y 좌표 반전

            % 인덱스 클리핑
            x_idx = min(max(x_idx, 1), 100);
            y_idx = min(max(y_idx, 1), 100);

            mapMatrix(y_idx, x_idx) = 1;
        end
    end
end

== matlab function Day4_5_Scenario_1/MATLAB Function2 ==
  settings: sampleTime=0.1
  data: traffic_info input; obstacle_list output
function obstacle_list = add_obstacle_(traffic_info)
    % 차량 사이즈
    car_w = 2.48;            % 전폭
    car_l = 11.5;            % 전장

    % 장애물 파라미터
    r = car_w / 2 + 2;       % 각 원의 반지름 (1.24 + 2)
    n_circles = 10;          % 각 차량당 원 개수
    interval = car_l / n_circles;  % 원 간격

    % 최대 장애물 개수
    max_obs = 70;
    obstacle_list = zeros(max_obs, 3);  % [x, y, r]

    % === 데이터 복원 ===
    % 데이터가 직렬화된 벡터 형태로 들어오는 경우 처리
    if size(traffic_info, 2) == 1
        % 데이터를 3열 형태로 변환
        n = length(traffic_info) / 3;
        if mod(length(traffic_info), 3) == 0
            % 직렬 데이터를 [N x 3] 행렬로 변환
            latest_data = reshape(traffic_info, 3, n)';  % [N x 3]
            %disp('Reconstructed Data:');
            %disp(latest_data);  % 디버그 출력
        else
            warning('Invalid data length for traffic_info');
            return;
        end
    else
        latest_data = traffic_info;
    end

    % === 데이터 유효성 검사 ===
    if isempty(latest_data) || size(latest_data, 2) < 3
        warning('Latest data is empty or has incorrect dimensions');
        return;
    end

    % 중복 제거: unique 함수 사용 가능 여부 확인
    if size(latest_data, 1) > 1
        % unique 함수로 중복 좌표 제거
        [~, unique_indices] = unique(latest_data(:, 1:2), 'rows', 'stable');
        unique_data = latest_data(unique_indices, :);
    else
        % 데이터가 하나만 있는 경우 그대로 사용
        unique_data = latest_data;
    end

    % 입력 데이터 유효성 검사 및 reshape 처리
    unique_data = reshape(unique_data, [], 3);  % [N x 3]
    [n_rows, ~] = size(unique_data);

    % 장애물 좌표 생성
    count = 0;
    for i = 1:n_rows
        x_head = unique_data(i, 1);
        y_head = unique_data(i, 2);
        yaw = unique_data(i, 3);  % 각도(rad)

        % Yaw 값 검증
        if isnan(yaw) || ~isfinite(yaw)
            yaw = 0;
        end

        % 장애물 생성 (차량의 길이 방향으로)
        for j = 0:n_circles-1
            dx = cos(yaw) * (j * interval);
            dy = sin(yaw) * (j * interval);
            xc = x_head + dx;
            yc = y_head + dy;

            count = count + 1;
            if count <= max_obs
                obstacle_list(count, :) = [xc, yc, r];
            else
                break;
            end
        end
    end

    % 디버그: 결과 확인
    %disp('Generated Obstacle List:');
    %disp(obstacle_list);
end

== matlab function Day4_5_Scenario_1/Function-Call Subsystem1/MATLAB Function4 ==
  settings: sampleTime=0.05
  data: poly_coeff input; lateral_error output; velocity input; lookahead_time input; x_lookahead output
function [lateral_error, x_lookahead] = compute_lateral_error(poly_coeff, velocity, lookahead_time)
    
    % Lookahead 지점 계산
    x_lookahead = velocity * lookahead_time;
    % 경로 상의 lookahead 지점에서의 y값 계산
    y_desired = polyval(poly_coeff, x_lookahead);

    % lateral error : 차량 y=0 위치와 경로 y_desired의 차이
    lateral_error = y_desired;
end

== matlab function Day4_5_Scenario_1/Function-Call Subsystem1/MATLAB Function4  ==
  settings: sampleTime=0.05
  data: path input; local_waypoints_ output; vehicle_position input; head input
function local_waypoints_ = global_to_local_waypoints(path, vehicle_position, head)
    %#codegen
    % 글로벌 경로를 로컬 경로로 변환해주는 함수
    % path : [x, y, yaw] (경로 점들)
    % vehicle_position : [Ego_Global_X, Ego_Global_Y]
    % head : Ego_Yaw (rad)
    % 출력: 로컬 좌표 (x_local, y_local, yaw_local)

    % 최대 경로 점 개수 설정
    max_points = 100;

    % 초기화
    local_waypoints_ = NaN(max_points, 3);  % 고정 크기 배열

    % 차량 위치 및 헤딩 추출
    ego_x = vehicle_position(1);
    ego_y = vehicle_position(2);
    ego_yaw = head;

    % 회전 행렬 생성 (글로벌→로컬 변환)
    R = [cos(-ego_yaw) -sin(-ego_yaw); 
         sin(-ego_yaw)  cos(-ego_yaw)];

    count = int32(0);  % 경로 점 개수

    % 각 경로 포인트에 대해 변환 수행
    for i = 1:min(size(path, 1), max_points)
        % 글로벌 좌표에서 차량까지의 상대 위치
        dx = path(i, 1) - ego_x;  % X 좌표 차이
        dy = path(i, 2) - ego_y;  % Y 좌표 차이

        % 회전 변환 적용
        local_pos = R * [dx; dy];
        
        % Yaw 변환: 로컬 좌표계에서의 Yaw
        global_yaw = path(i, 3);
        local_yaw = wrapToPi(global_yaw - ego_yaw);  % 로컬 yaw 변환

        % 차량으로부터 waypoint까지의 거리
        distance = sqrt(local_pos(1)^2 + local_pos(2)^2);

        % 첫 번째 유효 경로 점 저장 (x > 0인 첫 포인트)
        if count == 0 && local_pos(1) > 0
            count = count + 1;
            local_waypoints_(count, :) = [local_pos(1), local_pos(2), local_yaw];
        end
        
        % 고정 크기 초과 방지
        if count < max_points
            count = count + 1;
            local_waypoints_(count, :) = [local_pos(1), local_pos(2), local_yaw];
        else
            warning('Maximum number of waypoints reached.');
            break;
        end
    end

    % 남은 부분을 NaN으로 채움
    if count < max_points
        local_waypoints_((count+1):max_points, :) = NaN;
    end
end

== matlab function Day4_5_Scenario_1/Function-Call Subsystem1/MATLAB Function5 ==
  settings: sampleTime=0.05
  data: local_waypoints input; poly_coeff output
function poly_coeff = fit_polynomial_to_waypoints(local_waypoints)
    % waypoint를 curve fitting 한 다항식 계수 반환
    % input: 로컬 좌표 웨이포인트
    % output: 다항식 계수 (3차)

    % 웨이포인트 추출
    x_points = local_waypoints(:, 1);  % 로컬 x 좌표
    y_points = local_waypoints(:, 2);  % 로컬 y 좌표

    % 유효한 웨이포인트만 사용 (x 좌표가 양수인 것만)
    valid_indices = x_points > 0;
    x_valid = x_points(valid_indices);
    y_valid = y_points(valid_indices);

    % 웨이포인트가 충분한지 확인
    if length(x_valid) < 4
        % 웨이포인트가 부족하면 직선 경로 반환
        poly_coeff = [0, 0, 0, 0];  % y = 0 (직선)
    else
        % 3차 다항식 피팅 (y = ax^3 + bx^2 + cx + d)
        poly_coeff = polyfit(x_valid, y_valid, 3);
    end
end

== matlab function Day4_5_Scenario_1/Function-Call Subsystem1/MATLAB Function2 ==
  settings: sampleTime=0.05
  data: currPoseRear input; DesiredAx output; ego_v input; target_velocity input; goalPose input; stopFlag output; target_velocity output
function [DesiredAx,stopFlag,target_velocity] = longitudinal_goal_controller(currPoseRear, ego_v,target_velocity,goalPose)
%▴ 종방향 속도 제어 및 목표 도달 확인
% Inputs:
%   currPoseRear: [x_rear; y_rear; psi] (후륜축 기준)
%   v           : 속도 (m/s)
%   goalPose    : [x_goal; y_goal; psi_goal]
% Outputs:
%   DesiredAx   : 원하는 가속도 (m/s^2)
%   stopFlag    : 목표 도달 시 true

    persistent Kp Kd dt prev_error
  if isempty(Kp)
    % — PD 게인 설정 (필요에 따라 조정하세요) —
    Kp = 1.8;    % 비례 이득
    Kd = 0.1;    % 미분 이득
    % — 제어 업데이트 주기 (Simulink 샘플타임과 동일하게) —
    dt = 0.1;    % [s]
    % — previous error 초기화 —
    prev_error = target_velocity - ego_v;
  end

  % 1) 속도 오차
  error = target_velocity - ego_v;
  % 2) 오차 변화율 (미분항)
  derivative = (error - prev_error) / dt;
  % 3) PD 제어 법칙
  DesiredAx = Kp * error + Kd * derivative;
  % 4) 이전 오차 갱신
  prev_error = error;


    %#codegen
    % 1) 위치·헤딩 오차 계산
    dx     = currPoseRear(1) - goalPose(1);
    dy     = currPoseRear(2) - goalPose(2);
    dist   = hypot(dx, dy);                                           % 거리 계산 :contentReference[oaicite:3]{index=3}
    yawErr = wrapToPi(goalPose(3) - currPoseRear(3));                 % –π~π 범위 :contentReference[oaicite:4]{index=4}

    % 2) 목표 도달 여부 판단 (Goal Checking in Parking Valet) :contentReference[oaicite:5]{index=5}
    posTol = 1.7;             % 위치 허용 오차 [m]
    yawTol = deg2rad(30);     % 헤딩 허용 오차 [rad]
    almostFlag = dist<12;
    distFlag = dist <= posTol;
    yawFlag = abs(yawErr) <= yawTol;
    stopFlag = distFlag && yawFlag;

    % 3) DesiredAx 계산
    if stopFlag
        DesiredAx = -1000;
        disp("stopFlag")% 도착 시 완전 정지
    elseif almostFlag
        target_velocity = 3;
        disp("almost goal")% 근접 시 제동 가속도
        error      = target_velocity - ego_v;
        derivative = (error - prev_error)/dt;
        DesiredAx  = Kp*error + Kd*derivative;
        prev_error = error;
    end
end

== matlab function Day4_5_Scenario_1/MATLAB Function3 ==
  data: start input; path output double size=[100, 3]; goal input; obstacle_list input double size=[70, 3]
function path = hybrid_astar_(start, goal, obstacle_list)
%#codegen

% 기본 파라미터 설정
R = 4;
Vx = 3;
delta_time_step = 1;
weight = 1.3;
space = [0, 100, -100, 0];
res_dijkstra = 1;

% 경로 배열 초기화 (고정 크기)
path = NaN(100, 3);  % 고정 크기 배열
path_count = int32(0);

% 구조체 초기화 함수
default_node = struct('position', zeros(1,3), 'heading', 0.0, 'g', 0.0, 'h', 0.0, 'f', 0.0, 'parent', int32(0));
open_list = repmat(default_node, 1, 100);
closed_list = repmat(default_node, 1, 10000);

% Dijkstra를 이용한 비용 맵 생성
cost_map = run_dijkstra(goal, obstacle_list, space, res_dijkstra);
start_node = create_node(int32(0), start);
goal_node = create_node(int32(0), goal);

% 초기화
open_list(1) = start_node;
open_count = int32(1);
closed_count = int32(0);

% Hybrid A* 알고리즘
while open_count > 0
    % 최저 비용 노드 선택
    f_values = arrayfun(@(n) n.f, open_list(1:open_count));
    [~, idx] = min(f_values);
    temp_node = open_list(idx);
    open_list(idx) = open_list(open_count);
    open_count = open_count - 1;
    closed_count = closed_count + 1;
    closed_list(closed_count) = temp_node;

    % 목표 도달 확인
    if isSamePosition(temp_node, goal_node, 5)
        % 역순으로 경로 저장
        idx = 1;  % 경로 인덱스 초기화
        while temp_node.parent > 0 && path_count < 100
            path_count = path_count + 1;
            % 경로를 역순으로 저장하여 고정 크기 유지
            path(path_count, :) = temp_node.position;
            parent_idx = temp_node.parent;
            temp_node = closed_list(parent_idx);  
            idx = idx + 1;
        end
        % 경로 배열 크기를 고정하여 반환
        if path_count < 100
            path((path_count+1):100, :) = NaN;  % 나머지 부분을 NaN으로 채움
        end
        return;
    end

    % 가능한 액션 생성 및 탐색
    actions = get_action(R, Vx, delta_time_step);
    for i = 1:size(actions, 1)
        yaw_rate = actions(i, 1);
        dt = actions(i, 2);
        new_pos = vehicle_move(temp_node.position, yaw_rate, dt, Vx);
        
        % 탐색 공간 확인 및 충돌 검사
        if isNotInSearchingSpace(new_pos, space), continue; end
        if collision_check(temp_node.position, yaw_rate, dt, obstacle_list, Vx, space), continue; end
        
        % 자식 노드 생성
        child_node = create_node(closed_count, new_pos);
        if any(arrayfun(@(n) isSamePosition(n, child_node, 5) && isSameYaw(n, child_node, 0.3), closed_list(1:closed_count))), continue; end
        
        % 비용 계산
        yaw_diff = abs(angdiff(temp_node.heading, child_node.heading));
        turn_penalty = 2 * yaw_diff;
        child_node.g = temp_node.g + Vx * dt + turn_penalty;
        child_node.h = heuristic(child_node, goal_node, cost_map, space, res_dijkstra);
        child_node.f = child_node.g + weight * child_node.h;

        % 중복 노드 체크
        skip = false;
        for j = 1:open_count
            temp_open = open_list(j);
            if isSamePosition(temp_open, child_node, 5) && child_node.f >= temp_open.f
                skip = true; break;
            end
        end
        if skip, continue; end

        % 오픈 리스트에 추가
        open_count = open_count + 1;
        open_list(open_count) = child_node;
    end
end
% 경로 크기 고정으로 반환
path = path(1:100, :);
end

% 노드 생성 함수
function node = create_node(parent, position)
    % 구조체 필드 초기화 고정
    node = struct('position', zeros(1,3), 'heading', 0.0, 'g', 0.0, 'h', 0.0, 'f', 0.0, 'parent', int32(parent));
    node.position = reshape(position, [1,3]);  % 강제로 크기 고정
    node.heading = position(3);
end

function h = heuristic(cur_node, goal_node, cost_map, space, res)
    gx = round((cur_node.position(1) - space(1)) / res) + 1;
    gy = round((cur_node.position(2) - space(3)) / res) + 1;
    [ny, nx] = size(cost_map);
    if gx < 1 || gx > nx || gy < 1 || gy > ny, h = 1e6; return; end
    cost_dijkstra = cost_map(gy, gx);
    dyaw = abs(angdiff(cur_node.heading, goal_node.heading));
    h = cost_dijkstra + 3 * dyaw;
end

function cost_map = run_dijkstra(goal, obstacle_list, space, res)
x_range = space(1):res:space(2);
y_range = space(3):res:space(4);
nx = length(x_range); ny = length(y_range);
cost_map = inf(ny, nx); visited = false(ny, nx);
gx = round((goal(1) - space(1)) / res) + 1;
gy = round((goal(2) - space(3)) / res) + 1;
cost_map(gy, gx) = 0;

% Preallocate the queue with a fixed size
q = zeros(10000, 2);
q_count = 1;
q(1, :) = [gx, gy];

while q_count > 0
    [~, idx] = min(cost_map(sub2ind(size(cost_map), q(1:q_count,2), q(1:q_count,1))));
    current = q(idx, :);
    q(idx, :) = q(q_count, :);
    q_count = q_count - 1;
    x = current(1); y = current(2);
    if visited(y, x), continue; end
    visited(y, x) = true;
    for dx = -1:1
        for dy = -1:1
            if dx == 0 && dy == 0, continue; end
            nx_ = x + dx; ny_ = y + dy;
            if nx_ < 1 || ny_ < 1 || nx_ > nx || ny_ > ny, continue; end
            px = space(1) + (nx_-1) * res;
            py = space(3) + (ny_-1) * res;
            in_collision = false;
            for k = 1:size(obstacle_list,1)
                if hypot(px - obstacle_list(k,1), py - obstacle_list(k,2)) < obstacle_list(k,3)
                    in_collision = true; break;
                end
            end
            if in_collision, continue; end
            cost = cost_map(y,x) + res * hypot(dx, dy);
            if cost < cost_map(ny_, nx_)
                cost_map(ny_, nx_) = cost;
                q_count = q_count + 1;
                q(q_count, :) = [nx_, ny_];
            end
        end
    end
end
end

function actions = get_action(R, Vx, delta_time_step)
    yaw_rate = Vx / R;
    distance_travel = Vx * delta_time_step;
    actions = [
        yaw_rate, delta_time_step, distance_travel;
       -yaw_rate, delta_time_step, distance_travel;
        yaw_rate/2, delta_time_step, distance_travel;
       -yaw_rate/2, delta_time_step, distance_travel;
        0.0, delta_time_step, distance_travel
    ];
end

function new_pos = vehicle_move(pos, yaw_rate, delta_time, Vx)
    x = pos(1); y = pos(2); yaw = pos(3);
    if abs(yaw_rate) > 1e-3
        R = Vx / yaw_rate;
        cx = x - R * sin(yaw);
        cy = y + R * cos(yaw);
        dtheta = yaw_rate * delta_time;
        x_new = cx + R * sin(yaw + dtheta);
        y_new = cy - R * cos(yaw + dtheta);
        yaw_new = yaw + dtheta;
    else
        x_new = x + Vx * delta_time * cos(yaw);
        y_new = y + Vx * delta_time * sin(yaw);
        yaw_new = yaw;
    end
    yaw_new = mod(yaw_new, 2*pi);
    new_pos = [x_new, y_new, yaw_new];
end

function is_collision = collision_check(pos, yaw_rate, dt, obs_list, Vx, space)
    new_pos = vehicle_move(pos, yaw_rate, dt, Vx);
    x = new_pos(1); y = new_pos(2);
    if x < space(1) || x > space(2) || y < space(3) || y > space(4)
        is_collision = true; disp('Out of boundary'); return;
    end
    is_collision = false;
    for i = 1:size(obs_list,1)
        dx = x - obs_list(i,1); dy = y - obs_list(i,2);
        if hypot(dx, dy) < obs_list(i,3)
            is_collision = true; 
            %disp('collision');
            return;
        end
    end
end

function same = isSamePosition(node1, node2, epsilon)
    dx = node1.position(1) - node2.position(1);
    dy = node1.position(2) - node2.position(2);
    same = hypot(dx, dy) < epsilon;
end

function same = isSameYaw(node1, node2, epsilon)
    dyaw = abs(wrapToPi(node1.heading - node2.heading));
    same = dyaw < epsilon;
end

function out = isNotInSearchingSpace(pos, space)
    x = pos(1); y = pos(2);
    out = ~(space(1) <= x && x <= space(2) && space(3) <= y && y <= space(4));
end

== matlab function Day4_5_Scenario_1/MATLAB Function4 ==
  settings: updateMethod=DISCRETE  sampleTime=0.05
  data: poly_coeff input; lateral_error output; velocity input; lookahead_time input; x_lookahead output
function [lateral_error, x_lookahead] = compute_lateral_error(poly_coeff, velocity, lookahead_time)
    
    % Lookahead 지점 계산
    x_lookahead = velocity * lookahead_time;
    % 경로 상의 lookahead 지점에서의 y값 계산
    y_desired = polyval(poly_coeff, x_lookahead);

    % lateral error : 차량 y=0 위치와 경로 y_desired의 차이
    lateral_error = y_desired;
end
